simulink model "Linear_IWP"  (R2022b)
settings: Solver=VariableStepAuto  StartTime=0.0  StopTime=20  RelTol=1e-3
undefined symbols (not defined in the file): a11_num, a21_num, a22_num, g, K_aug, mc_num
settings Model: Creator=User  LastModifiedBy=User

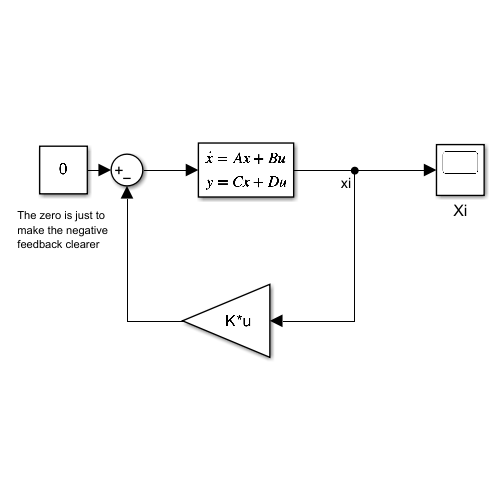
[thumbnail: Simulink's stored preview of the top-level diagram]
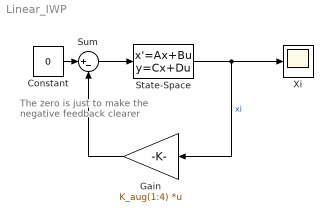
== system Linear_IWP ==
  note: The zero is just to
      | make the negative
      | feedback clearer
  Constant : Constant  Value=0
  Gain : Gain  Gain=K_aug(1:4)  Multiplication=Matrix(K*u)
  State-Space : StateSpace  A=[0 1 0 0; 0 0 1 0; 0 0 0 1; 0 0 0 0]  B=[0; 0; 0; 1]  C=eye(4)  D=[0; 0; 0; 0]  InitialCondition=[a22_num*pi/4 0 a11_num*(a22_num*a21_num)*mc_num*g*sin(pi/4) 0]  ContinuousStateAttributes='xi'
  Sum : Sum  Inputs=|+-
  Xi : Scope
  wires:
  Gain/1 -> Sum/2
  State-Space/1 -> Xi/1, Gain/1  "xi"
  Sum/1 -> State-Space/1
  Constant/1 -> Sum/1
